simulink model "Lorenz"  (R2020b)
settings: Solver=VariableStepAuto  StartTime=0.0  StopTime=50  RelTol=1e-3
libraries: simulink x1
settings Model: Creator=tian  LastModifiedBy=tian

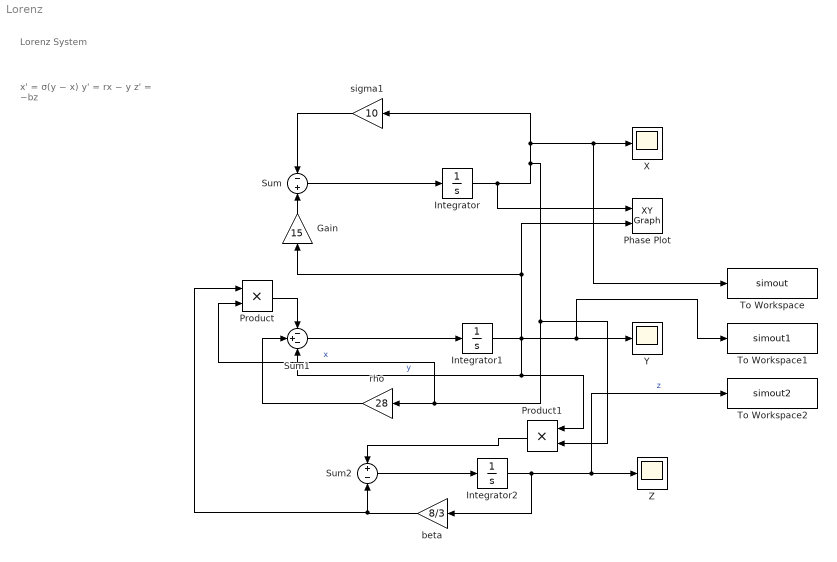
== system Lorenz ==
  note: x' = σ(y − x)
      | y' = rx − y
      | z' = −bz
  note: Lorenz System
  Gain : Gain  Gain=15
  Integrator : Integrator  InitialCondition=1
  Integrator1 : Integrator  InitialCondition=1
  Integrator2 : Integrator  InitialCondition=1
  Phase Plot : simulink/Sinks/XY Graph  xmin=-20  xmax=20  ymin=-20  ymax=20  st=0.01
  Product : Product
  Product1 : Product
  Sum : Sum  Inputs=-+
  Sum1 : Sum  Inputs=-+-
  Sum2 : Sum  Inputs=+-
  To Workspace : ToWorkspace  VariableName=simout  SampleTime=-1
  To Workspace1 : ToWorkspace  VariableName=simout1  SampleTime=-1
  To Workspace2 : ToWorkspace  VariableName=simout2  SampleTime=-1
  X : Scope
  Y : Scope
  Z : Scope
  beta : Gain  Gain=8/3
  rho : Gain  Gain=28
  sigma1 : Gain  Gain=10
  wires:
  sigma1/1 -> Sum/1
  Sum/1 -> Integrator/1
  Integrator1/1 -> Product1/1, Sum1/3, To Workspace1/1, Y/1, Gain/1, Phase Plot/2  "y"
  Product/1 -> Sum1/1
  Sum1/1 -> Integrator1/1
  rho/1 -> Sum1/2
  Integrator/1 -> Product1/2, Product/2, rho/1, sigma1/1, To Workspace/1, X/1, Phase Plot/1  "x"
  Product1/1 -> Sum2/1
  Sum2/1 -> Integrator2/1
  Integrator2/1 -> beta/1, To Workspace2/1, Z/1  "z"
  Gain/1 -> Sum/2
  beta/1 -> Product/1, Sum2/2
